simulink model "flightController"  (R2025b)
settings: Solver=ode3  StartTime=0  StopTime=TFinal  FixedStep=Ts  RelTol=1e-3  EnableMultiTasking=on
undefined symbols (not defined in the file): Controller, g, Ts, useTrueAlt, useTrueAtt, useTruePos, Vehicle
settings Model: Creator=The MathWorks, Inc.  LastModifiedBy=user
settings SolverCC: AlgebraicLoopSolver=TrustRegion  MinimalZcImpactIntegration=on
settings DataIOCC: LimitDataPoints=on  SaveFormat=Array  ReturnWorkspaceOutputs=off
settings OptimizationCC: BlockReduction=off  DefaultParameterBehavior=Inlined  BufferReuse=off  PassReuseOutputArgsThreshold=0.0
settings DebuggingCC: AlgebraicLoopMsg=none  ParameterPrecisionLossMsg=none  ParameterTunabilityLossMsg=error  BusObjectLabelMismatch=error  SFUnexpectedBacktrackingDiag=warning  SFNoUnconditionalDefaultTransitionDiag=warning  SFExecutionAtInitializationDiag=none  ArithmeticOperatorsInVariantConditions=warning
settings HardwareCC: ProdBitPerPointer=32.0  ProdBitPerSizeT=32.0  ProdBitPerPtrDiffT=32.0  ProdLargestAtomicInteger=Long  ProdWordSize=32.0  ProdHWDeviceType=ARM Compatible->ARM 9
settings ModelReferenceCC: EnableRefExpFcnMdlSchedulingChecks=on  ModelReferenceNumInstancesAllowed=Single  PropagateSignalLabelsOutOfModel=off
settings SFSimCC: SimUseLocalCustomCode=off  CustomCodeUndefinedFunction=UseInterfaceOnly
settings RTWCC: GenerateReport=on  RTWUseLocalCustomCode=off  LaunchReport=on  GPUComputeCapability=3.5
settings CodeAppCC: ForceParamTrailComments=on  MaxIdLength=63.0  OperatorAnnotations=on  StateflowObjectComments=on  MATLABSourceComments=on
settings GRTTargetCC: TargetLangStandard=C89/C90 (ANSI)  SubcomponentCodeInterfacePackaging=Nonreusable function
settings ConfigComp: CovMetricSettings=dw  CovSaveCumulativeToWorkspaceVar=on  CovSaveSingleToWorkspaceVar=on  CovExternalEMLEnable=off  CovSFcnEnable=off

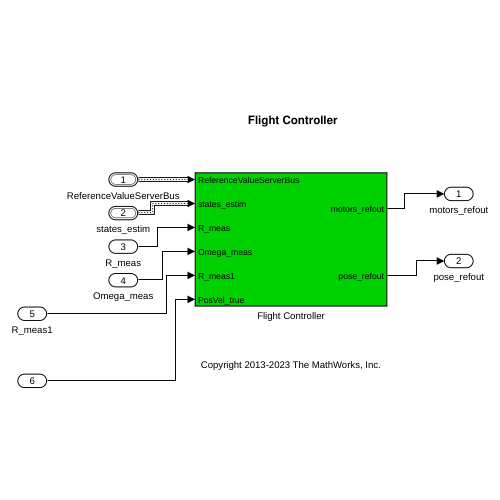
[thumbnail: Simulink's stored preview of the top-level diagram]
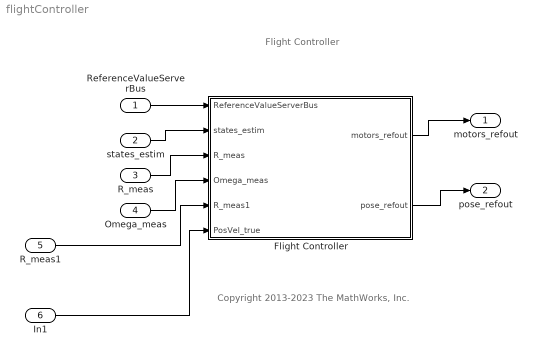
== system flightController ==
  note: Flight Controller
  note: Copyright 2013-2023 The MathWorks, Inc.
  ReferenceValueServerBus : Inport  OutDataTypeStr=Bus: CommandBus  BusOutputAsStruct=on
  states_estim : Inport  Port=2  OutDataTypeStr=Bus: statesEstim_t  BusOutputAsStruct=on
  R_meas : Inport  Port=3  PortDimensions=[3 3]
  Omega_meas : Inport  Port=4  PortDimensions=[3 1]
  R_meas1 : Inport  Port=5  PortDimensions=[3 3]
  In1 : Inport  Port=6
  Flight Controller : Subsystem
  motors_refout : Outport  VectorParamsAs1DForOutWhenUnconnected=off
  pose_refout : Outport  Port=2  VectorParamsAs1DForOutWhenUnconnected=off
  wires:
  ReferenceValueServerBus/1 -> Flight Controller/1(ReferenceValueServerBus)
  states_estim/1 -> Flight Controller/2(states_estim)
  Flight Controller/2(pose_refout) -> pose_refout/1
  Flight Controller/1(motors_refout) -> motors_refout/1
  R_meas/1 -> Flight Controller/3(R_meas)
  Omega_meas/1 -> Flight Controller/4(Omega_meas)
  R_meas1/1 -> Flight Controller/5(R_meas1)
  In1/1 -> Flight Controller/6(PosVel_true)

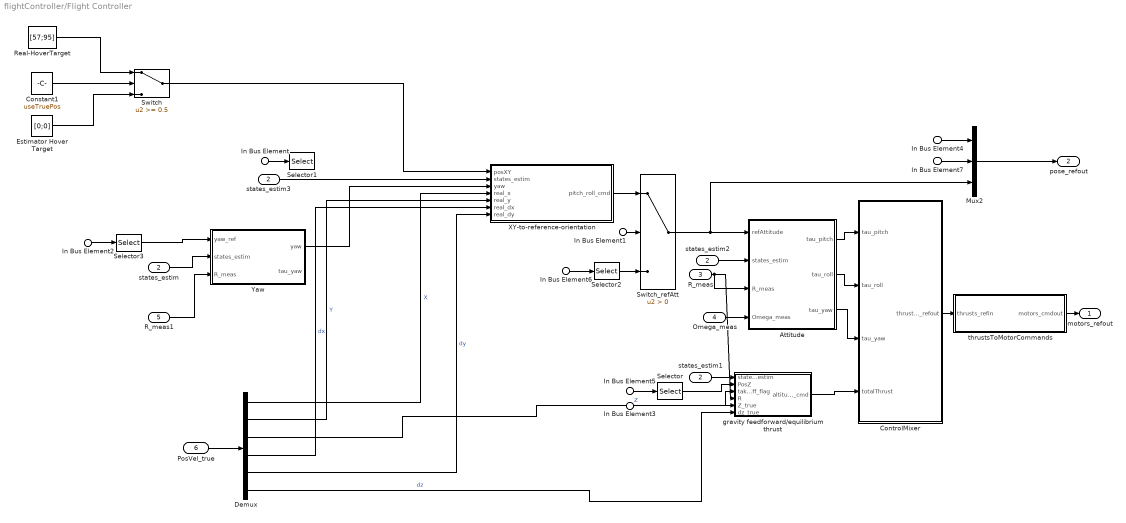
== system flightController/Flight Controller ==
  In Bus Element1 : Inport  PortName=ReferenceValueServerBus  Element=controlModePosVSOrient
  In Bus Element : Inport  PortName=ReferenceValueServerBus  Element=pos_ref
  In Bus Element4 : Inport  PortName=ReferenceValueServerBus  Element=pos_ref
  In Bus Element5 : Inport  PortName=ReferenceValueServerBus  Element=pos_ref
  In Bus Element2 : Inport  PortName=ReferenceValueServerBus  Element=orient_ref
  In Bus Element6 : Inport  PortName=ReferenceValueServerBus  Element=orient_ref
  In Bus Element7 : Inport  PortName=ReferenceValueServerBus  Element=orient_ref
  In Bus Element3 : Inport  PortName=ReferenceValueServerBus  Element=takeoff_flag
  states_estim : Inport  Port=2
  R_meas : Inport  Port=3  PortDimensions=[3 3]
  Omega_meas : Inport  Port=4  PortDimensions=[3 1]
  R_meas1 : Inport  Port=5  PortDimensions=[3 3]
  PosVel_true : Inport  Port=6
  Attitude : Subsystem
  Constant1 : Constant  Value=useTruePos
  ControlMixer : Subsystem
  Demux : Demux  Outputs=6
  Estimator Hover Target : Constant  Value=[0;0]  OutDataTypeStr=double
  Mux2 : Mux  Inputs=3
  Real-HoverTarget : Constant  Value=[57;95]  OutDataTypeStr=double
  Selector : Selector  InputPortWidth=3  IndexOptions=Index vector (dialog)  Indices=3  OutputSizes=1
  Selector1 : Selector  InputPortWidth=3  IndexOptions=Index vector (dialog)  Indices=[1 2]  OutputSizes=1
  Selector2 : Selector  InputPortWidth=3  IndexOptions=Index vector (dialog)  Indices=[2 3]  OutputSizes=1
  Selector3 : Selector  InputPortWidth=3  IndexOptions=Index vector (dialog)  Indices=1  OutputSizes=1
  Switch : Switch  Threshold=0.5  SaturateOnIntegerOverflow=off  InputSameDT=off
  Switch_refAtt : Switch  Criteria=u2 > Threshold  SaturateOnIntegerOverflow=off  InputSameDT=off
  XY-to-reference-orientation : Subsystem
  Yaw : Subsystem
  gravity feedforward/equilibrium thrust : Subsystem
  states_estim1 : InportShadow  Port=2
  states_estim2 : InportShadow  Port=2
  states_estim3 : InportShadow  Port=2
  thrustsToMotorCommands : Subsystem
  motors_refout : Outport  VectorParamsAs1DForOutWhenUnconnected=off
  pose_refout : Outport  Port=2  VectorParamsAs1DForOutWhenUnconnected=off
  wires:
  thrustsToMotorCommands/1(motors_cmdout) -> motors_refout/1
  In Bus Element1/1 -> Switch_refAtt/2
  XY-to-reference-orientation/1(pitch_roll_cmd) -> Switch_refAtt/1
  In Bus Element2/1 -> Selector3/1
  In Bus Element/1 -> Selector1/1
  Selector3/1 -> Yaw/1(yaw_ref)
  ControlMixer/1(thrusts_refout) -> thrustsToMotorCommands/1(thrusts_refin)
  In Bus Element3/1 -> gravity feedforward/equilibrium thrust/3(takeoff_flag)
  states_estim/1 -> Yaw/2(states_estim)
  Switch_refAtt/1 -> Mux2/3, Attitude/1(refAttitude)
  Yaw/1(yaw) -> XY-to-reference-orientation/3(yaw)
  gravity feedforward/equilibrium thrust/1(altitude_cmd) -> ControlMixer/4(totalThrust)
  Mux2/1 -> pose_refout/1
  Attitude/1(tau_pitch) -> ControlMixer/1(tau_pitch)
  Attitude/2(tau_roll) -> ControlMixer/2(tau_roll)
  states_estim1/1 -> gravity feedforward/equilibrium thrust/1(states_estim)
  states_estim2/1 -> Attitude/2(states_estim)
  In Bus Element4/1 -> Mux2/1
  Selector/1 -> gravity feedforward/equilibrium thrust/2(PosZ)
  In Bus Element5/1 -> Selector/1
  In Bus Element6/1 -> Selector2/1
  Selector2/1 -> Switch_refAtt/3
  In Bus Element7/1 -> Mux2/2
  R_meas/1 -> gravity feedforward/equilibrium thrust/4(R), Attitude/3(R_meas)
  Omega_meas/1 -> Attitude/4(Omega_meas)
  R_meas1/1 -> Yaw/3(R_meas)
  PosVel_true/1 -> Demux/1
  Demux/1 -> XY-to-reference-orientation/4(real_x)  "X"
  Demux/2 -> XY-to-reference-orientation/5(real_y)  "Y"
  Demux/3 -> gravity feedforward/equilibrium thrust/5(Z_true)  "Z"
  Demux/5 -> XY-to-reference-orientation/7(real_dy)  "dy"
  Demux/6 -> gravity feedforward/equilibrium thrust/6(dz_true)  "dz"
  states_estim3/1 -> XY-to-reference-orientation/2(states_estim)
  Attitude/3(tau_yaw) -> ControlMixer/3(tau_yaw)
  Demux/4 -> XY-to-reference-orientation/6(real_dx)  "dx"
  Constant1/1 -> Switch/2
  Estimator Hover Target/1 -> Switch/3
  Real-HoverTarget/1 -> Switch/1
  Switch/1 -> XY-to-reference-orientation/1(posXY)

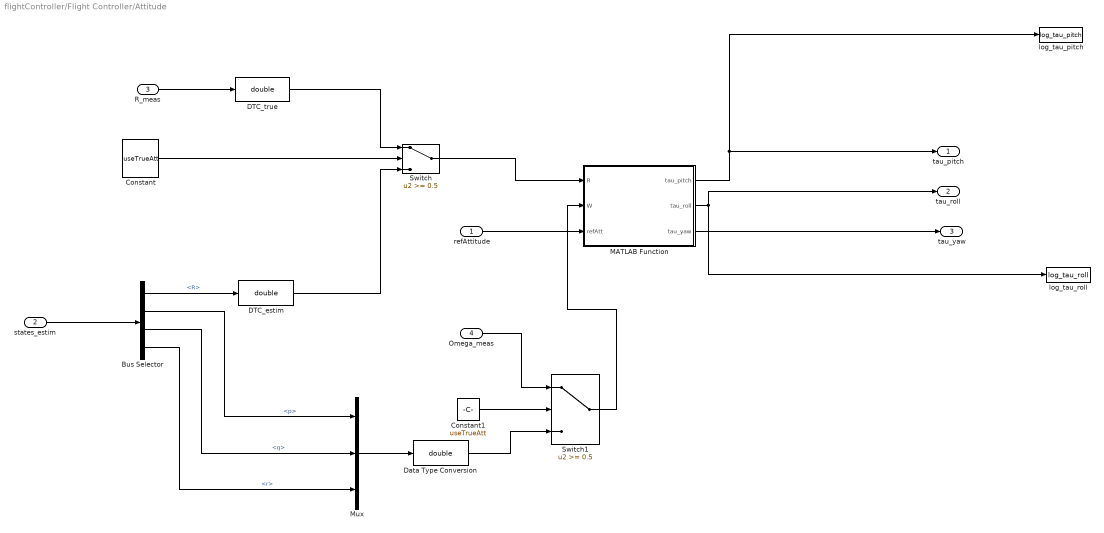
== system flightController/Flight Controller/Attitude ==
  refAttitude : Inport
  states_estim : Inport  Port=2
  R_meas : Inport  Port=3  PortDimensions=[3 3]
  Omega_meas : Inport  Port=4  PortDimensions=[3 1]
  Bus Selector : BusSelector  OutputSignals=R,p,q,r
  Constant : Constant  Value=useTrueAtt
  Constant1 : Constant  Value=useTrueAtt
  DTC_estim : DataTypeConversion  OutDataTypeStr=double  SaturateOnIntegerOverflow=off  RndMeth=Floor
  DTC_true : DataTypeConversion  OutDataTypeStr=double  SaturateOnIntegerOverflow=off  RndMeth=Floor
  Data Type Conversion : DataTypeConversion  OutDataTypeStr=double  SaturateOnIntegerOverflow=off  RndMeth=Floor
  MATLAB Function : MATLAB Function  TreatAsAtomicUnit=on
  Mux : Mux  Inputs=3
  Switch : Switch  Threshold=0.5  SaturateOnIntegerOverflow=off  InputSameDT=off
  Switch1 : Switch  Threshold=0.5  SaturateOnIntegerOverflow=off  InputSameDT=off
  log_tau_pitch : ToWorkspace  VariableName=log_tau_pitch  SaveFormat=Timeseries  SampleTime=-1
  log_tau_roll : ToWorkspace  VariableName=log_tau_roll  SaveFormat=Timeseries  SampleTime=-1
  tau_pitch : Outport  VectorParamsAs1DForOutWhenUnconnected=off
  tau_roll : Outport  Port=2  VectorParamsAs1DForOutWhenUnconnected=off
  tau_yaw : Outport  Port=3
  wires:
  refAttitude/1 -> MATLAB Function/3(refAtt)
  MATLAB Function/1(tau_pitch) -> log_tau_pitch/1, tau_pitch/1
  MATLAB Function/2(tau_roll) -> tau_roll/1, log_tau_roll/1
  MATLAB Function/3(tau_yaw) -> tau_yaw/1
  states_estim/1 -> Bus Selector/1
  R_meas/1 -> DTC_true/1
  DTC_true/1 -> Switch/1
  Constant/1 -> Switch/2
  Bus Selector/1 -> DTC_estim/1  "<R>"
  DTC_estim/1 -> Switch/3
  Switch/1 -> MATLAB Function/1(R)
  Bus Selector/2 -> Mux/1  "<p>"
  Bus Selector/3 -> Mux/2  "<q>"
  Bus Selector/4 -> Mux/3  "<r>"
  Mux/1 -> Data Type Conversion/1
  Omega_meas/1 -> Switch1/1
  Constant1/1 -> Switch1/2
  Data Type Conversion/1 -> Switch1/3
  Switch1/1 -> MATLAB Function/2(W)

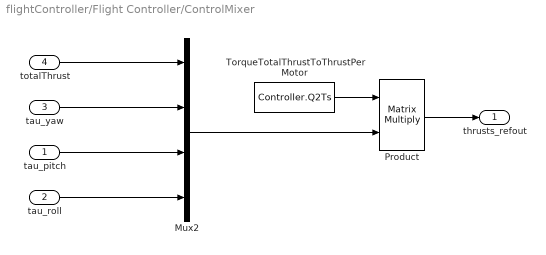
== system flightController/Flight Controller/ControlMixer ==
  tau_pitch : Inport
  tau_roll : Inport  Port=2
  tau_yaw : Inport  Port=3
  totalThrust : Inport  Port=4
  Mux2 : Mux
  Product : Product  Multiplication=Matrix(*)  RndMeth=Zero
  TorqueTotalThrustToThrustPerMotor : Constant  Value=Controller.Q2Ts  OutDataTypeStr=single
  thrusts_refout : Outport  VectorParamsAs1DForOutWhenUnconnected=off
  wires:
  Product/1 -> thrusts_refout/1
  tau_roll/1 -> Mux2/4
  tau_pitch/1 -> Mux2/3
  tau_yaw/1 -> Mux2/2
  totalThrust/1 -> Mux2/1
  TorqueTotalThrustToThrustPerMotor/1 -> Product/1
  Mux2/1 -> Product/2

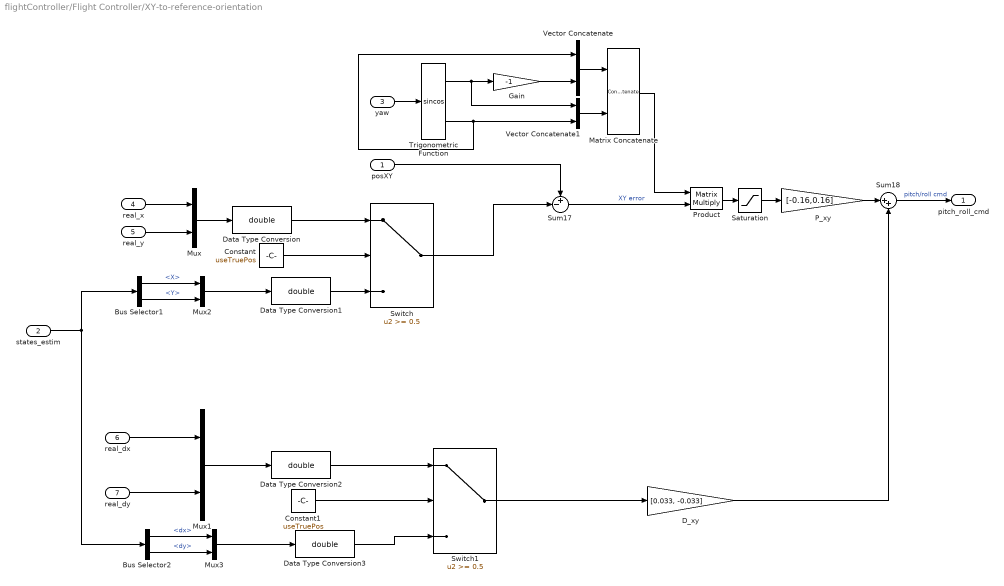
== system flightController/Flight Controller/XY-to-reference-orientation ==
  posXY : Inport
  states_estim : Inport  Port=2
  yaw : Inport  Port=3
  real_x : Inport  Port=4
  real_y : Inport  Port=5
  real_dx : Inport  Port=6
  real_dy : Inport  Port=7
  Bus Selector1 : BusSelector  OutputSignals=X,Y
  Bus Selector2 : BusSelector  OutputSignals=dx,dy
  Constant : Constant  Value=useTruePos
  Constant1 : Constant  Value=useTruePos
  D_xy : Gain  Gain=[0.033, -0.033]  ParamDataTypeStr=single  OutDataTypeStr=single  SaturateOnIntegerOverflow=on
  Data Type Conversion{,1..3} (4 alike) : DataTypeConversion  OutDataTypeStr=double  SaturateOnIntegerOverflow=off  RndMeth=Floor
  Gain : Gain  Gain=-1
  Matrix Concatenate : Concatenate  Mode=Multidimensional array  ConcatenateDimension=2
  Mux{,1..3} (4 alike) : Mux  Inputs=2
  P_xy : Gain  Gain=[-0.16,0.16]  ParamDataTypeStr=single  OutDataTypeStr=single  SaturateOnIntegerOverflow=on
  Product : Product  Multiplication=Matrix(*)  OutDataTypeStr=single  RndMeth=Zero
  Saturation : Saturate  UpperLimit=3  LowerLimit=-3  OutDataTypeStr=single
  Sum17 : Sum  Inputs=+-|  AccumDataTypeStr=single
  Sum18 : Sum  Inputs=|++  OutDataTypeStr=single  AccumDataTypeStr=single  SaturateOnIntegerOverflow=on
  Switch : Switch  Threshold=0.5  SaturateOnIntegerOverflow=off  InputSameDT=off
  Switch1 : Switch  Threshold=0.5  SaturateOnIntegerOverflow=off  InputSameDT=off
  Trigonometric Function : Trigonometry  Operator=sincos
  Vector Concatenate : Concatenate
  Vector Concatenate1 : Concatenate
  pitch_roll_cmd : Outport  VectorParamsAs1DForOutWhenUnconnected=off
  wires:
  yaw/1 -> Trigonometric Function/1
  Saturation/1 -> P_xy/1
  P_xy/1 -> Sum18/1
  Sum17/1 -> Product/2  "XY error"
  posXY/1 -> Sum17/1
  states_estim/1 -> Bus Selector1/1, Bus Selector2/1
  Sum18/1 -> pitch_roll_cmd/1  "pitch/roll cmd"
  D_xy/1 -> Sum18/2
  Product/1 -> Saturation/1
  Trigonometric Function/1 -> Gain/1, Vector Concatenate1/1
  Trigonometric Function/2 -> Vector Concatenate1/2, Vector Concatenate/1
  Gain/1 -> Vector Concatenate/2
  Vector Concatenate/1 -> Matrix Concatenate/1
  Vector Concatenate1/1 -> Matrix Concatenate/2
  Matrix Concatenate/1 -> Product/1
  real_x/1 -> Mux/1
  real_y/1 -> Mux/2
  real_dx/1 -> Mux1/1
  real_dy/1 -> Mux1/2
  Mux/1 -> Data Type Conversion/1
  Data Type Conversion/1 -> Switch/1
  Constant/1 -> Switch/2
  Bus Selector1/1 -> Mux2/1  "<X>"
  Bus Selector1/2 -> Mux2/2  "<Y>"
  Mux2/1 -> Data Type Conversion1/1
  Data Type Conversion1/1 -> Switch/3
  Switch/1 -> Sum17/2
  Mux1/1 -> Data Type Conversion2/1
  Data Type Conversion2/1 -> Switch1/1
  Constant1/1 -> Switch1/2
  Bus Selector2/1 -> Mux3/1  "<dx>"
  Bus Selector2/2 -> Mux3/2  "<dy>"
  Mux3/1 -> Data Type Conversion3/1
  Data Type Conversion3/1 -> Switch1/3
  Switch1/1 -> D_xy/1

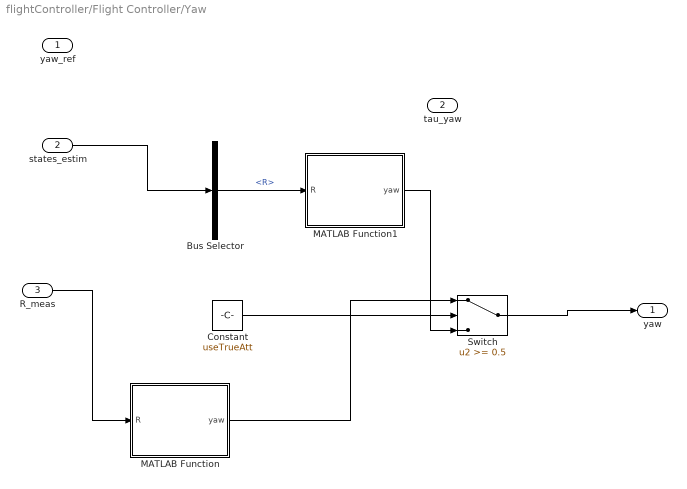
== system flightController/Flight Controller/Yaw ==
  yaw_ref : Inport
  states_estim : Inport  Port=2
  R_meas : Inport  Port=3
  Bus Selector : BusSelector  OutputSignals=R
  Constant : Constant  Value=useTrueAtt
  MATLAB Function : MATLAB Function  TreatAsAtomicUnit=on
  MATLAB Function1 : MATLAB Function  TreatAsAtomicUnit=on
  Switch : Switch  Threshold=0.5  SaturateOnIntegerOverflow=off  InputSameDT=off
  yaw : Outport  VectorParamsAs1DForOutWhenUnconnected=off
  tau_yaw : Outport  Port=2  VectorParamsAs1DForOutWhenUnconnected=off
  wires:
  R_meas/1 -> MATLAB Function/1(R)
  states_estim/1 -> Bus Selector/1
  Bus Selector/1 -> MATLAB Function1/1(R)  "<R>"
  MATLAB Function/1(yaw) -> Switch/1
  Constant/1 -> Switch/2
  MATLAB Function1/1(yaw) -> Switch/3
  Switch/1 -> yaw/1

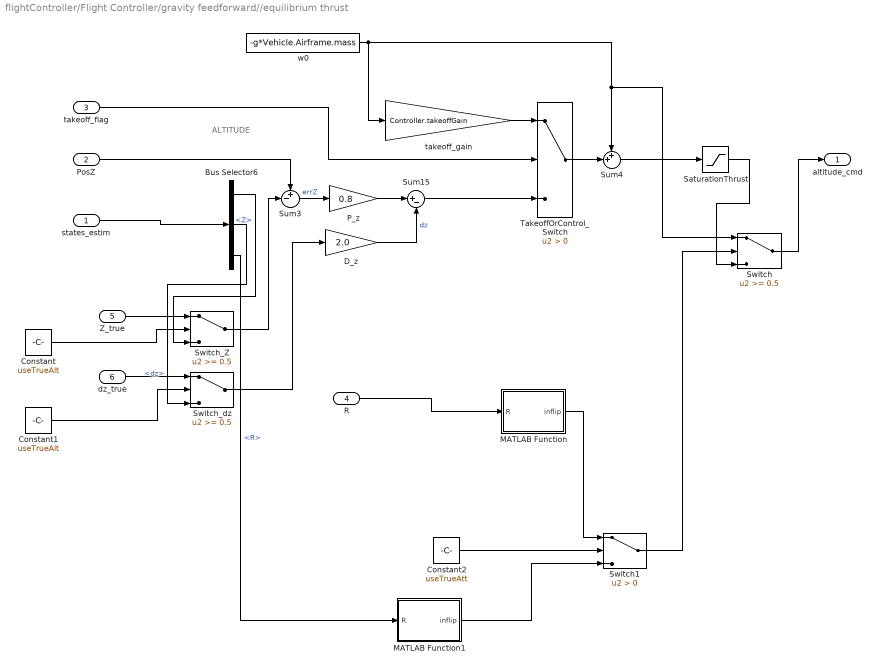
== system flightController/Flight Controller/gravity feedforward//equilibrium thrust ==
  note: ALTITUDE
  states_estim : Inport
  PosZ : Inport  Port=2
  takeoff_flag : Inport  Port=3
  R : Inport  Port=4
  Z_true : Inport  Port=5  OutDataTypeStr=double
  dz_true : Inport  Port=6  OutDataTypeStr=double
  Bus Selector6 : BusSelector  OutputSignals=Z,dz,R
  Constant : Constant  Value=useTrueAlt
  Constant1 : Constant  Value=useTrueAlt
  Constant2 : Constant  Value=useTrueAtt
  D_z : Gain  Gain=2.0  ParamDataTypeStr=single  OutDataTypeStr=single  SaturateOnIntegerOverflow=on
  MATLAB Function : MATLAB Function  TreatAsAtomicUnit=on
  MATLAB Function1 : MATLAB Function  TreatAsAtomicUnit=on
  P_z : Gain  Gain=0.8  ParamDataTypeStr=single  OutDataTypeStr=single  SaturateOnIntegerOverflow=on
  SaturationThrust : Saturate  UpperLimit=4*Controller.totalThrustMaxRelative*Controller.motorsThrustPerMotorMax  LowerLimit=-4*Controller.totalThrustMaxRelative*Controller.motorsThrustPerMotorMax  OutDataTypeStr=single
  Sum15 : Sum  Inputs=|+-  OutDataTypeStr=single  AccumDataTypeStr=single  SaturateOnIntegerOverflow=on
  Sum3 : Sum  Inputs=+-|  OutDataTypeStr=single  AccumDataTypeStr=single  SaturateOnIntegerOverflow=on
  Sum4 : Sum  Inputs=++|  OutDataTypeStr=single  AccumDataTypeStr=single  SaturateOnIntegerOverflow=on
  Switch : Switch  Threshold=0.5  SaturateOnIntegerOverflow=off  InputSameDT=off
  Switch1 : Switch  Criteria=u2 > Threshold  SaturateOnIntegerOverflow=off  InputSameDT=off
  Switch_Z : Switch  Threshold=0.5  SaturateOnIntegerOverflow=off  InputSameDT=off
  Switch_dz : Switch  Threshold=0.5  SaturateOnIntegerOverflow=off  InputSameDT=off
  TakeoffOrControl_Switch : Switch  Criteria=u2 > Threshold  SaturateOnIntegerOverflow=off  InputSameDT=off
  takeoff_gain : Gain  Gain=Controller.takeoffGain  ParamDataTypeStr=single  OutDataTypeStr=single  SaturateOnIntegerOverflow=on
  w0 : Constant  Value=-g*Vehicle.Airframe.mass  OutDataTypeStr=single  SampleTime=Ts
  altitude_cmd : Outport  VectorParamsAs1DForOutWhenUnconnected=off
  wires:
  Sum3/1 -> P_z/1  "errZ"
  w0/1 -> Switch/1, Sum4/1, takeoff_gain/1
  D_z/1 -> Sum15/2  "dz"
  takeoff_gain/1 -> TakeoffOrControl_Switch/1
  takeoff_flag/1 -> TakeoffOrControl_Switch/2
  PosZ/1 -> Sum3/1
  P_z/1 -> Sum15/1
  states_estim/1 -> Bus Selector6/1
  Sum15/1 -> TakeoffOrControl_Switch/3
  Sum4/1 -> SaturationThrust/1
  TakeoffOrControl_Switch/1 -> Sum4/2
  SaturationThrust/1 -> Switch/3
  Switch/1 -> altitude_cmd/1
  R/1 -> MATLAB Function/1(R)
  Z_true/1 -> Switch_Z/1
  dz_true/1 -> Switch_dz/1
  Constant/1 -> Switch_Z/2
  Constant1/1 -> Switch_dz/2
  Bus Selector6/1 -> Switch_Z/3  "<Z>"
  Bus Selector6/2 -> Switch_dz/3  "<dz>"
  Switch_Z/1 -> Sum3/2
  Switch_dz/1 -> D_z/1
  Bus Selector6/3 -> MATLAB Function1/1(R)  "<R>"
  Constant2/1 -> Switch1/2
  MATLAB Function1/1(inflip) -> Switch1/3
  MATLAB Function/1(inflip) -> Switch1/1
  Switch1/1 -> Switch/2

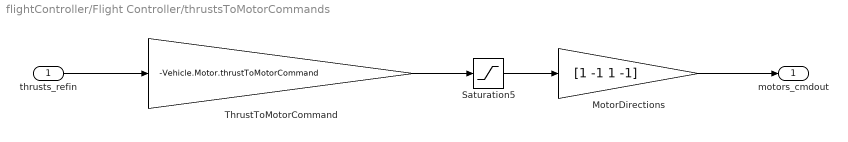
== system flightController/Flight Controller/thrustsToMotorCommands ==
  thrusts_refin : Inport
  MotorDirections : Gain  Gain=[1 -1 1 -1]
  Saturation5 : Saturate  UpperLimit=Vehicle.Motor.maxLimit  LowerLimit=Vehicle.Motor.minLimit
  ThrustToMotorCommand : Gain  Gain=-Vehicle.Motor.thrustToMotorCommand
  motors_cmdout : Outport  VectorParamsAs1DForOutWhenUnconnected=off
  wires:
  Saturation5/1 -> MotorDirections/1
  MotorDirections/1 -> motors_cmdout/1
  ThrustToMotorCommand/1 -> Saturation5/1
  thrusts_refin/1 -> ThrustToMotorCommand/1

== matlab function flightController/Flight Controller/Yaw/MATLAB Function ==
  data: R input; yaw output
function yaw = R2yaw(R)
Rb2e = double(R)';
yaw  = atan2(Rb2e(2,1), Rb2e(1,1));
end

== matlab function flightController/Flight Controller/Attitude/MATLAB Function ==
  data: R input; tau_pitch output; W input; tau_roll output; refAtt input; tau_yaw output
function [tau_pitch, tau_roll, tau_yaw] = GeometricController(R, W, refAtt)

    % ===== 고정 파라미터 =====
    kR = 0.06;   kW = 0.006;
    J  = diag([5.82857e-5, 7.16914e-5, 1e-4]);
    a_max    = 394;      % rad/s^2   = tau_max/Jyy, 포화시 각감속도
    tau_max  = 0.0282;   % N*m       = 2L(fmax-fmin)
    R33_exit = 0.707;    % cos(45deg), 해제 기울기 (추력예산 33% 확보)

    R_b2e = double(R.');
    Wd    = double(W);
    R33   = R_b2e(3,3);

    % ===== 물리량 =====
    w_tilt = hypot(Wd(1), Wd(2));                  % 기울임 각속도 (yaw 제외)
    theta  = acos(min(1, max(-1, R33)));           % 기울기 0..pi
    w_crit = sqrt(2*a_max*max(0, pi - theta));     % 플립 완주 판정선
    w_sat  = tau_max / kW;                         % D항 포화 경계 (~4.7)

    % ===== 플립 모드 (래치 + 히스테리시스) =====
    persistent inFlip
    if isempty(inFlip)
        inFlip = false;
    end

    if ~inFlip
        % 진입: 90° 넘었거나, 최대제동으로도 못 멈추는 각속도
        inFlip = (R33 < 0) || (w_tilt > w_crit);
    else
        % 해제: 45° 안으로 복귀 AND 제어기가 선형영역 복귀
        inFlip = ~( (R33 > R33_exit) && (w_tilt < w_sat) );
    end

    % ===== R_des =====
    if inFlip
        R_des = eye(3);                            % 플립 중: 수평 고정
    else
        p = double(refAtt(1));
        r = double(refAtt(2));
        Ry = [cos(p) 0 sin(p); 0 1 0; -sin(p) 0 cos(p)];
        Rx = [1 0 0; 0 cos(r) -sin(r); 0 sin(r) cos(r)];
        R_des = Ry*Rx;
    end

    % ===== 기하 제어 =====
    W_des = [0; 0; 0];
    eR  = vee(0.5*(R_des.'*R_b2e - R_b2e.'*R_des));
    eW  = Wd - R_b2e.'*R_des*W_des;
    % ===== tilt-torsion 분리 =====
    if inFlip
        w_yaw = 0.0;
    else
        w_yaw = max(0, min(1, R33));   % 복귀 구간: 기울기 비례로 완만 복원
    end
    eR(3) = w_yaw * eR(3);

    tau = -kR*eR - kW*eW + cross(Wd, J*Wd);

    tau_pitch = single(tau(2));
    tau_roll  = single(tau(1));
    tau_yaw   = single(tau(3));
end

function v = vee(M)
    v = [M(3,2); M(1,3); M(2,1)];
end

== matlab function flightController/Flight Controller/gravity feedforward//equilibrium thrust/MATLAB Function ==
  data: R input; inflip output
function inflip = flipWindow(R)
    inflip = double(R(3,3) <= 0);   % 기울기 90° 넘으면(R(3,3)이 0 이하) 끔
end

== matlab function flightController/Flight Controller/Yaw/MATLAB Function1 ==
  data: R input; yaw output
function yaw = R2yaw(R)
Rb2e = double(R)';
yaw  = atan2(Rb2e(2,1), Rb2e(1,1));
end

== matlab function flightController/Flight Controller/gravity feedforward//equilibrium thrust/MATLAB Function1 ==
  data: R input; inflip output
function inflip = flipWindow(R)
    inflip = double(R(3,3) <= 0);   % 기울기 90° 넘으면(R(3,3)이 0 이하) 끔
end
